simulink model "F16Block"  (R2017a)
settings: Solver=VariableStepAuto  StartTime=0.0  StopTime=400  FixedStep=delta_T  RelTol=1e-3  EnableMultiTasking=on
values from neighbouring files (symbols this model uses):
  trim_control = [xu(2);xu(4);xu(5)]    [trim_F16.m]
  trim_state = xu(1:12)    [trim_F16.m]
  trim_thrust = xu(13)    [trim_F16.m]
undefined symbols (not defined in the file or in its folder): DisAil_1, DisAil_2, DisAil_3, DisEle_1, DisEle_2, DisEle_3, DisRud_1, DisRud_2, DisRud_3, fi_flag_Simulink
libraries: F16_Actuator_Library x9
settings Model: ExtModeAutoUpdateStatusClock=off  Creator=keviczky  LastModifiedBy=wagneda1
settings DataIOCC: Decimation=50  SaveFormat=Array  SignalLoggingName=sigsOut
settings OptimizationCC: BooleanDataType=off
settings DebuggingCC: SaveWithParameterizedLinksMsg=none  UnderspecifiedInitializationDetection=Classic  MergeDetectMultiDrivingBlocksExec=none  SignalResolutionControl=TryResolveAllWithWarning  MultiTaskDSMMsg=warning  MultiTaskCondExecSysMsg=none
settings HardwareCC: ProdBitPerPointer=32  ProdBitPerSizeT=32  ProdBitPerPtrDiffT=32  ProdLargestAtomicFloat=None  ProdIntDivRoundTo=Undefined  ProdEndianess=Unspecified  ProdWordSize=32  ProdHWDeviceType=32-bit Generic  TargetUnknown=on
settings ModelReferenceCC: PropagateSignalLabelsOutOfModel=off
settings GRTTargetCC: TargetLangStandard=C89/C90 (ANSI)  CombineOutputUpdateFcns=off  GRTInterface=on
settings ConfigComp: CovMetricSettings=dw  CovHtmlReporting=on  CovSaveCumulativeToWorkspaceVar=on  CovSaveSingleToWorkspaceVar=on  CovExternalEMLEnable=off

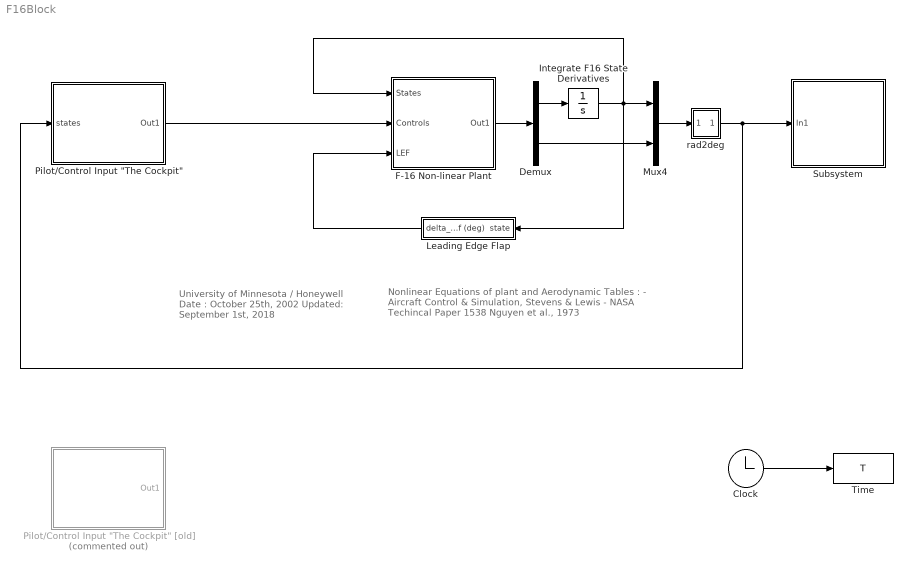
== system F16Block ==
  note: University of Minnesota / Honeywell
      | Date : October 25th, 2002
      | Updated: September 1st, 2018
  note: Nonlinear Equations of plant and Aerodynamic Tables :
      | - Aircraft Control & Simulation, Stevens & Lewis
      | - NASA Techincal Paper 1538 Nguyen et al., 1973
  Clock : Clock
      settings: Decimation=50
  Demux : Demux  Outputs=[12 6]
  F-16 Non-linear Plant : Subsystem
      mask Display: image('f16thumb.jpg')
  Integrate F16 State Derivatives : Integrator  InitialCondition=trim_state
  Leading Edge Flap : Subsystem
  Mux4 : Mux  Inputs=2
  "Pilot/Control Input \"The Cockpit\"" : Subsystem
      mask Display: image('f16cockpit.jpg')
  "Pilot/Control Input \"The Cockpit\" [old]" : Subsystem  Commented=on
      mask Display: image(imread('f16cockpit.jpg'))
  Subsystem : Subsystem
      mask Display: image('f16output.jpg')
  Time : ToWorkspace  VariableName=T  SampleTime=-1
      settings: Decimation=100
  rad2deg : Subsystem
  wires:
  Mux4/1 -> rad2deg/1(In1)
  Demux/1 -> Integrate F16 State Derivatives/1
  Demux/2 -> Mux4/2
  "Pilot/Control Input \"The Cockpit\""/1(Out1) -> F-16 Non-linear Plant/2(Controls)
  Leading Edge Flap/1(delta_lef (deg)) -> F-16 Non-linear Plant/3(LEF)
  F-16 Non-linear Plant/1(Out1) -> Demux/1
  Integrate F16 State Derivatives/1 -> Mux4/1, Leading Edge Flap/1(state), F-16 Non-linear Plant/1(States)
  Clock/1 -> Time/1
  rad2deg/1(Out1) -> "Pilot/Control Input \"The Cockpit\""/1(states), Subsystem/1(In1)

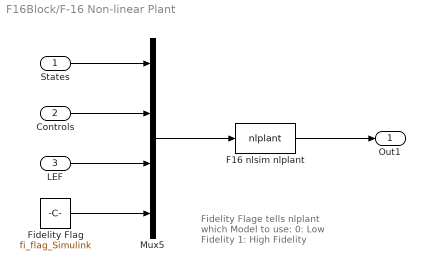
== system F16Block/F-16 Non-linear Plant ==
  note: Fidelity Flage tells nlplant
      | which Model to use:
      | 0: Low Fidelity
      | 1: High Fidelity
  States : Inport
  Controls : Inport  Port=2
  LEF : Inport  Port=3
  F16 nlsim nlplant : MATLABFcn  MATLABFcn=nlplant  OutputDimensions=18  OutputSignalType=real
  Fidelity Flag : Constant  Value=fi_flag_Simulink
  Mux5 : Mux  Inputs=[12 4 1 1]
  Out1 : Outport
  wires:
  Mux5/1 -> F16 nlsim nlplant/1
  F16 nlsim nlplant/1 -> Out1/1
  Fidelity Flag/1 -> Mux5/4
  LEF/1 -> Mux5/3
  Controls/1 -> Mux5/2
  States/1 -> Mux5/1

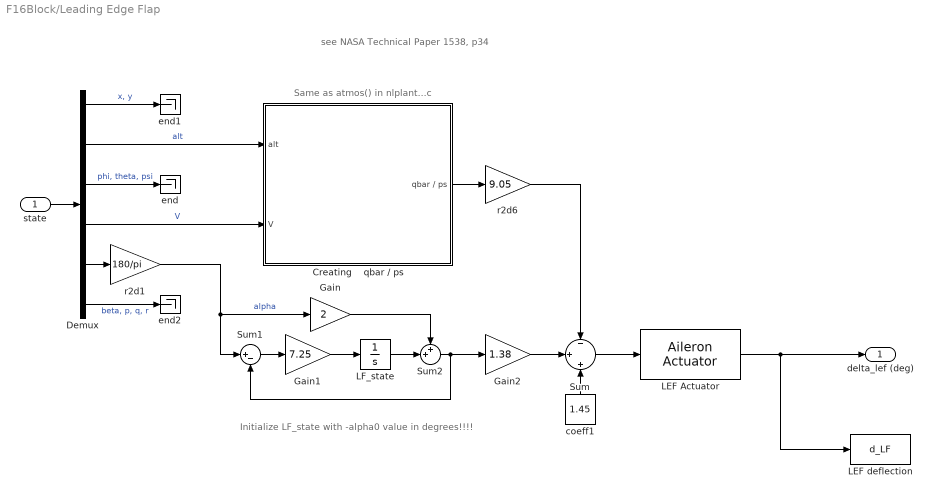
== system F16Block/Leading Edge Flap ==
  note: see NASA Technical Paper 1538, p34
  note: Same as atmos() in nlplant...c
  note: Initialize LF_state with -alpha0 value in degrees!!!!
  state : Inport
  Creating    qbar / ps : Subsystem
  Demux : Demux  Outputs=[2,1,3,1,1,4]
  Gain : Gain  Gain=2  SaturateOnIntegerOverflow=on  OutDataTypeStr=Inherit: Same as input  ParamDataTypeStr=Inherit: Same as input
  Gain1 : Gain  Gain=7.25  SaturateOnIntegerOverflow=on  OutDataTypeStr=Inherit: Same as input  ParamDataTypeStr=Inherit: Same as input
  Gain2 : Gain  Gain=1.38  SaturateOnIntegerOverflow=on  OutDataTypeStr=Inherit: Same as input  ParamDataTypeStr=Inherit: Same as input
  LEF Actuator : F16_Actuator_Library/Aileron Actuator
      link override Command Saturation: UpperLimit=25  LowerLimit=0
      link override Gain: Gain=1/0.136
      link override "Integrator ": InitialCondition=dLEF
      link override Rate Saturation: UpperLimit=25  LowerLimit=-25
  LEF deflection : ToWorkspace  VariableName=d_LF  SampleTime=-1
      settings: Decimation=100
  LF_state : Integrator  InitialCondition=-trim_state(8)*180/pi
  Sum : Sum  Inputs=-|+|+  SaturateOnIntegerOverflow=on  InputSameDT=on  OutDataTypeStr=Inherit: Same as first input
  Sum1 : Sum  Inputs=|+-  SaturateOnIntegerOverflow=on  InputSameDT=on  OutDataTypeStr=Inherit: Same as first input
  Sum2 : Sum  Inputs=++|  SaturateOnIntegerOverflow=on  InputSameDT=on  OutDataTypeStr=Inherit: Same as first input
  coeff1 : Constant  Value=1.45
  end : Terminator
  end1 : Terminator
  end2 : Terminator
  r2d1 : Gain  Gain=180/pi  SaturateOnIntegerOverflow=on  OutDataTypeStr=Inherit: Same as input  ParamDataTypeStr=Inherit: Same as input
  r2d6 : Gain  Gain=9.05  SaturateOnIntegerOverflow=on  OutDataTypeStr=Inherit: Same as input  ParamDataTypeStr=Inherit: Same as input
  delta_lef (deg) : Outport
  wires:
  LEF Actuator/1 -> LEF deflection/1, delta_lef (deg)/1
  Sum/1 -> LEF Actuator/1
  Demux/3 -> end/1  "phi, theta, psi"
  state/1 -> Demux/1
  Sum1/1 -> Gain1/1
  Gain1/1 -> LF_state/1
  Gain/1 -> Sum2/1
  Gain2/1 -> Sum/2
  Demux/1 -> end1/1  "x, y"
  Demux/5 -> r2d1/1
  Demux/6 -> end2/1  "beta, p, q, r"
  coeff1/1 -> Sum/3
  Sum2/1 -> Sum1/2, Gain2/1
  LF_state/1 -> Sum2/2
  r2d1/1 -> Sum1/1, Gain/1  "alpha"
  Demux/4 -> Creating    qbar / ps/2(V)  "V"
  Creating    qbar / ps/1(qbar / ps) -> r2d6/1
  r2d6/1 -> Sum/1
  Demux/2 -> Creating    qbar / ps/1(alt)  "alt"

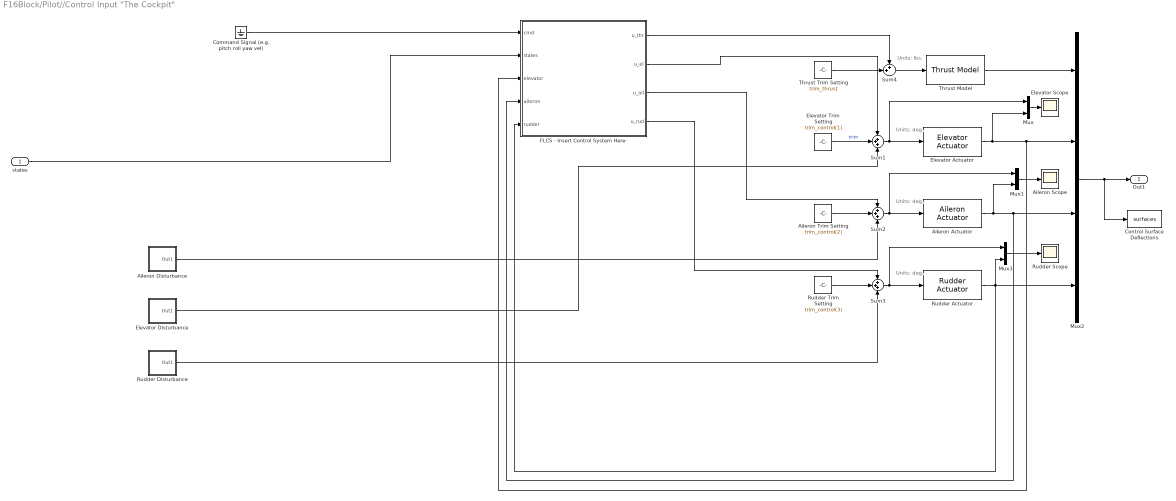
== system F16Block/Pilot//Control Input "The Cockpit" ==
  note: Units: lbs.
  note: Units: deg.
  note: Units: deg.
  note: Units: deg.
  states : Inport
  Aileron Actuator : F16_Actuator_Library/Aileron Actuator
  Aileron Scope : Scope
  Aileron Disturbance : Subsystem
  Aileron Trim Setting : Constant  Value=trim_control(2)
  Command Signal (e.g. pitch roll yaw vel) : Ground
  Control Surface Deflections : ToWorkspace  VariableName=surfaces  SampleTime=-1
      settings: Decimation=100
  Elevator Actuator : F16_Actuator_Library/Elevator Actuator
  Elevator Scope : Scope
  Elevator Disturbance : Subsystem
  Elevator Trim Setting : Constant  Value=trim_control(1)  VectorParams1D=off
  FLCS - Insert Control System Here- : Subsystem
  Mux : Mux  Inputs=2
  Mux1 : Mux  Inputs=2
  Mux2 : Mux
  Mux3 : Mux  Inputs=2
  Rudder Actuator : F16_Actuator_Library/Rudder Actuator
  Rudder Scope : Scope
  Rudder Disturbance : Subsystem
  Rudder Trim Setting : Constant  Value=trim_control(3)
  Sum1 : Sum  Inputs=+++  SaturateOnIntegerOverflow=on  InputSameDT=on  OutDataTypeStr=Inherit: Same as first input
  Sum2 : Sum  Inputs=+++  SaturateOnIntegerOverflow=on  InputSameDT=on  OutDataTypeStr=Inherit: Same as first input
  Sum3 : Sum  Inputs=+++  SaturateOnIntegerOverflow=on  InputSameDT=on  OutDataTypeStr=Inherit: Same as first input
  Sum4 : Sum  Inputs=++|  SaturateOnIntegerOverflow=on  InputSameDT=on  OutDataTypeStr=Inherit: Same as first input
  Thrust Model : F16_Actuator_Library/Thrust Model
  Thrust Trim Setting : Constant  Value=trim_thrust
  Out1 : Outport
  wires:
  Thrust Model/1 -> Mux2/1
  Sum1/1 -> Mux/1, Elevator Actuator/1
  Elevator Trim Setting/1 -> Sum1/2  "trim"
  Sum2/1 -> Mux1/1, Aileron Actuator/1
  Aileron Trim Setting/1 -> Sum2/2
  Sum3/1 -> Mux3/1, Rudder Actuator/1
  Rudder Trim Setting/1 -> Sum3/2
  Mux2/1 -> Out1/1, Control Surface Deflections/1
  Elevator Actuator/1 -> FLCS - Insert Control System Here-/3(elevator), Mux2/2, Mux/2
  Aileron Actuator/1 -> FLCS - Insert Control System Here-/4(aileron), Mux2/3, Mux1/2
  Rudder Actuator/1 -> Mux2/4, Mux3/2, FLCS - Insert Control System Here-/5(rudder)
  Mux/1 -> Elevator Scope/1
  Mux1/1 -> Aileron Scope/1
  Mux3/1 -> Rudder Scope/1
  Sum4/1 -> Thrust Model/1
  Thrust Trim Setting/1 -> Sum4/2
  Elevator Disturbance/1(Out1) -> Sum1/3
  Aileron Disturbance/1(Out1) -> Sum2/3
  Rudder Disturbance/1(Out1) -> Sum3/3
  states/1 -> FLCS - Insert Control System Here-/2(states)
  Command Signal (e.g. pitch roll yaw vel)/1 -> FLCS - Insert Control System Here-/1(cmd)
  FLCS - Insert Control System Here-/1(u_thr) -> Sum4/1
  FLCS - Insert Control System Here-/2(u_el) -> Sum1/1
  FLCS - Insert Control System Here-/3(u_ail) -> Sum2/1
  FLCS - Insert Control System Here-/4(u_rud) -> Sum3/1

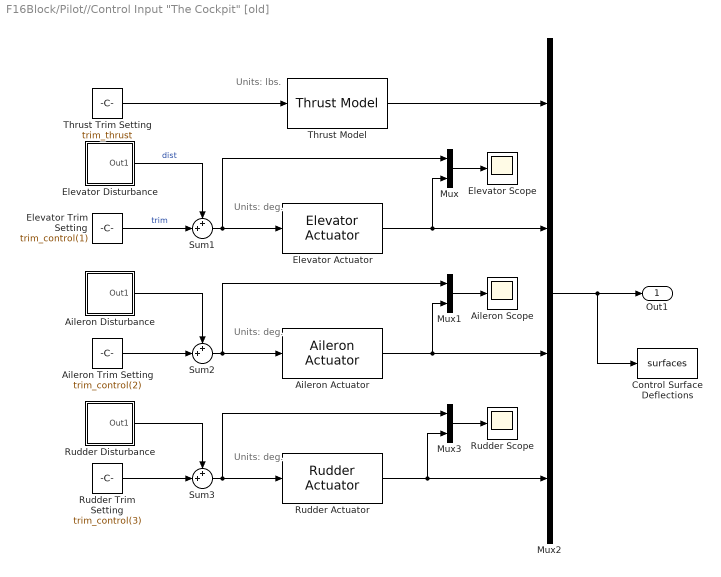
== system F16Block/Pilot//Control Input "The Cockpit" [old] ==
  note: Units: lbs.
  note: Units: deg.
  note: Units: deg.
  note: Units: deg.
  Aileron Actuator : F16_Actuator_Library/Aileron Actuator
  Aileron Scope : Scope
  Aileron Disturbance : Subsystem
  Aileron Trim Setting : Constant  Value=trim_control(2)
  Control Surface Deflections : ToWorkspace  VariableName=surfaces  SampleTime=-1
      settings: Decimation=100
  Elevator Actuator : F16_Actuator_Library/Elevator Actuator
  Elevator Scope : Scope
  Elevator Disturbance : Subsystem
  Elevator Trim Setting : Constant  Value=trim_control(1)  VectorParams1D=off
  Mux : Mux  Inputs=2
  Mux1 : Mux  Inputs=2
  Mux2 : Mux
  Mux3 : Mux  Inputs=2
  Rudder Actuator : F16_Actuator_Library/Rudder Actuator
  Rudder Scope : Scope
  Rudder Disturbance : Subsystem
  Rudder Trim Setting : Constant  Value=trim_control(3)
  Sum1 : Sum  Inputs=++|  SaturateOnIntegerOverflow=on  InputSameDT=on  OutDataTypeStr=Inherit: Same as first input
  Sum2 : Sum  Inputs=++|  SaturateOnIntegerOverflow=on  InputSameDT=on  OutDataTypeStr=Inherit: Same as first input
  Sum3 : Sum  Inputs=++|  SaturateOnIntegerOverflow=on  InputSameDT=on  OutDataTypeStr=Inherit: Same as first input
  Thrust Model : F16_Actuator_Library/Thrust Model
  Thrust Trim Setting : Constant  Value=trim_thrust
  Out1 : Outport
  wires:
  Thrust Model/1 -> Mux2/1
  Sum1/1 -> Mux/1, Elevator Actuator/1
  Elevator Trim Setting/1 -> Sum1/2  "trim"
  Sum2/1 -> Mux1/1, Aileron Actuator/1
  Aileron Trim Setting/1 -> Sum2/2
  Aileron Disturbance/1(Out1) -> Sum2/1
  Elevator Disturbance/1(Out1) -> Sum1/1  "dist"
  Sum3/1 -> Mux3/1, Rudder Actuator/1
  Rudder Disturbance/1(Out1) -> Sum3/1
  Rudder Trim Setting/1 -> Sum3/2
  Mux2/1 -> Out1/1, Control Surface Deflections/1
  Elevator Actuator/1 -> Mux2/2, Mux/2
  Aileron Actuator/1 -> Mux2/3, Mux1/2
  Rudder Actuator/1 -> Mux2/4, Mux3/2
  Mux/1 -> Elevator Scope/1
  Mux1/1 -> Aileron Scope/1
  Mux3/1 -> Rudder Scope/1
  Thrust Trim Setting/1 -> Thrust Model/1

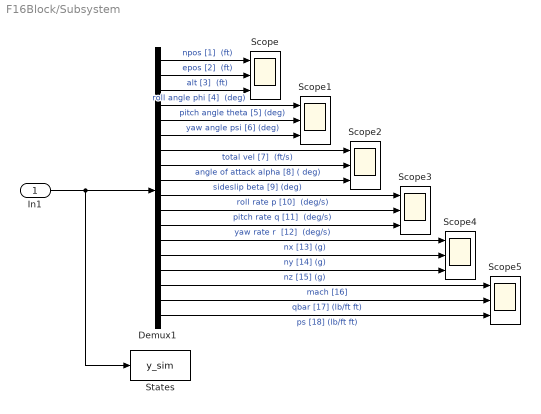
== system F16Block/Subsystem ==
  In1 : Inport
  Demux1 : Demux  Outputs=18
  Scope{,1..5} (6 alike) : Scope  NumInputPorts=3
  States : ToWorkspace  VariableName=y_sim  SampleTime=-1
      settings: Decimation=100
  wires:
  Demux1/1 -> Scope/1  "npos [1]  (ft)"
  Demux1/2 -> Scope/2  "epos [2]  (ft)"
  Demux1/3 -> Scope/3  "alt [3]  (ft)"
  Demux1/5 -> Scope1/2  "pitch angle theta [5] (deg)"
  Demux1/6 -> Scope1/3  "yaw angle psi [6] (deg)"
  Demux1/7 -> Scope2/1  "total vel [7]  (ft/s)"
  Demux1/8 -> Scope2/2  "angle of attack alpha [8] ( deg)"
  Demux1/9 -> Scope2/3  "sideslip beta [9] (deg)"
  Demux1/10 -> Scope3/1  "roll rate p [10]  (deg/s)"
  Demux1/11 -> Scope3/2  "pitch rate q [11]  (deg/s)"
  Demux1/12 -> Scope3/3  "yaw rate r  [12]  (deg/s)"
  Demux1/13 -> Scope4/1  "nx [13] (g)"
  Demux1/14 -> Scope4/2  "ny [14] (g)"
  Demux1/15 -> Scope4/3  "nz [15] (g)"
  Demux1/4 -> Scope1/1  "roll angle phi [4]  (deg)"
  Demux1/16 -> Scope5/1  "mach [16]"
  Demux1/17 -> Scope5/2  "qbar [17] (lb/ft ft)"
  Demux1/18 -> Scope5/3  "ps [18] (lb/ft ft)"
  In1/1 -> Demux1/1, States/1

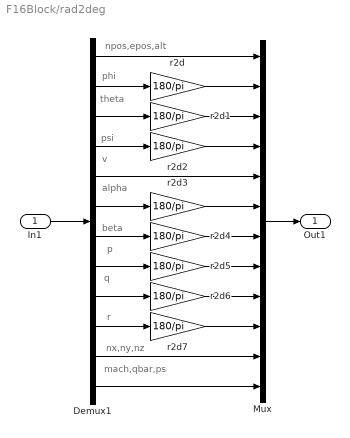
== system F16Block/rad2deg ==
  note: npos,epos,alt
  note: phi
  note: theta
  note: psi
  note: v
  note: alpha
  note: beta
  note: p
  note: q
  note: r
  note: nx,ny,nz
  note: mach,qbar,ps
  In1 : Inport
  Demux1 : Demux  Outputs=[3 1 1 1 1 1 1 1 1 1 3 3]
  Mux : Mux  Inputs=[3 1 1 1 1 1 1 1 1 1 3 3]
  r2d{,1..7} (8 alike) : Gain  Gain=180/pi  SaturateOnIntegerOverflow=on  OutDataTypeStr=Inherit: Same as input  ParamDataTypeStr=Inherit: Same as input
  Out1 : Outport
  wires:
  In1/1 -> Demux1/1
  Demux1/2 -> r2d/1
  Demux1/3 -> r2d1/1
  Demux1/4 -> r2d2/1
  Demux1/1 -> Mux/1
  Demux1/5 -> Mux/5
  r2d2/1 -> Mux/4
  r2d1/1 -> Mux/3
  r2d/1 -> Mux/2
  Demux1/6 -> r2d3/1
  Demux1/7 -> r2d4/1
  Demux1/8 -> r2d5/1
  Demux1/9 -> r2d6/1
  Demux1/10 -> r2d7/1
  r2d4/1 -> Mux/7
  r2d5/1 -> Mux/8
  r2d6/1 -> Mux/9
  r2d7/1 -> Mux/10
  Mux/1 -> Out1/1
  Demux1/11 -> Mux/11
  Demux1/12 -> Mux/12
  r2d3/1 -> Mux/6

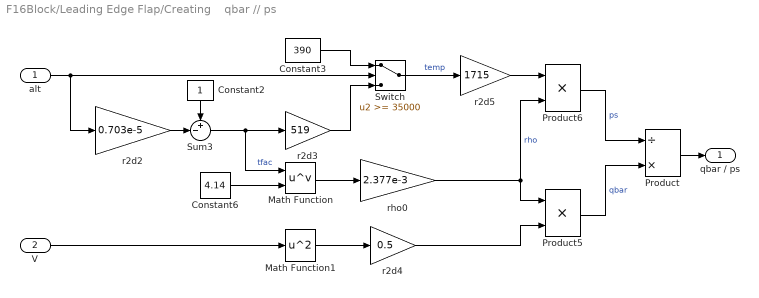
== system F16Block/Leading Edge Flap/Creating    qbar // ps ==
  alt : Inport
  V : Inport  Port=2
  Constant2 : Constant
  Constant3 : Constant  Value=390
  Constant6 : Constant  Value=4.14
  Math Function : Math  Operator=pow  SaturateOnIntegerOverflow=on
  Math Function1 : Math  Operator=square  SaturateOnIntegerOverflow=on
  Product : Product  Inputs=/*  SaturateOnIntegerOverflow=on  InputSameDT=on  OutDataTypeStr=Inherit: Same as first input
  Product5 : Product  Inputs=**  SaturateOnIntegerOverflow=on  InputSameDT=on  OutDataTypeStr=Inherit: Same as first input
  Product6 : Product  Inputs=**  SaturateOnIntegerOverflow=on  InputSameDT=on  OutDataTypeStr=Inherit: Same as first input
  Sum3 : Sum  Inputs=+-|  SaturateOnIntegerOverflow=on  InputSameDT=on  OutDataTypeStr=Inherit: Same as first input
  Switch : Switch  Threshold=35000  SaturateOnIntegerOverflow=on  InputSameDT=on
  r2d2 : Gain  Gain=0.703e-5  SaturateOnIntegerOverflow=on  OutDataTypeStr=Inherit: Same as input  ParamDataTypeStr=Inherit: Same as input
  r2d3 : Gain  Gain=519  SaturateOnIntegerOverflow=on  OutDataTypeStr=Inherit: Same as input  ParamDataTypeStr=Inherit: Same as input
  r2d4 : Gain  Gain=0.5  SaturateOnIntegerOverflow=on  OutDataTypeStr=Inherit: Same as input  ParamDataTypeStr=Inherit: Same as input
  r2d5 : Gain  Gain=1715  SaturateOnIntegerOverflow=on  OutDataTypeStr=Inherit: Same as input  ParamDataTypeStr=Inherit: Same as input
  rho0 : Gain  Gain=2.377e-3  SaturateOnIntegerOverflow=on  OutDataTypeStr=Inherit: Same as input  ParamDataTypeStr=Inherit: Same as input
  qbar / ps : Outport
  wires:
  alt/1 -> r2d2/1, Switch/2
  Sum3/1 -> Math Function/1, r2d3/1  "tfac"
  Constant3/1 -> Switch/1
  r2d3/1 -> Switch/3
  Constant6/1 -> Math Function/2
  rho0/1 -> Product5/1, Product6/2  "rho"
  Math Function1/1 -> r2d4/1
  r2d2/1 -> Sum3/2
  Constant2/1 -> Sum3/1
  Math Function/1 -> rho0/1
  r2d4/1 -> Product5/2
  Switch/1 -> r2d5/1  "temp"
  r2d5/1 -> Product6/1
  Product6/1 -> Product/1  "ps"
  Product5/1 -> Product/2  "qbar"
  Product/1 -> qbar / ps/1
  V/1 -> Math Function1/1

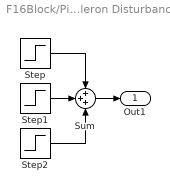
== system F16Block/Pilot//Control Input "The Cockpit"/Aileron Disturbance ==
  Step : Step  After=DisAil_1  SampleTime=0
  Step1 : Step  Time=3  After=DisAil_2  SampleTime=0
  Step2 : Step  Time=5  After=DisAil_3  SampleTime=0
  Sum : Sum  Inputs=+++  SaturateOnIntegerOverflow=on  InputSameDT=on  OutDataTypeStr=Inherit: Same as first input
  Out1 : Outport
  wires:
  Step1/1 -> Sum/2
  Step/1 -> Sum/1
  Step2/1 -> Sum/3
  Sum/1 -> Out1/1

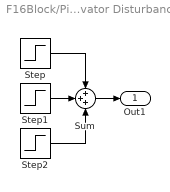
== system F16Block/Pilot//Control Input "The Cockpit"/Elevator Disturbance ==
  Step : Step  After=DisEle_1  SampleTime=0
  Step1 : Step  Time=3  After=DisEle_2  SampleTime=0
  Step2 : Step  Time=5  After=DisEle_3  SampleTime=0
  Sum : Sum  Inputs=+++  SaturateOnIntegerOverflow=on  InputSameDT=on  OutDataTypeStr=Inherit: Same as first input
  Out1 : Outport
  wires:
  Step1/1 -> Sum/2
  Step/1 -> Sum/1
  Step2/1 -> Sum/3
  Sum/1 -> Out1/1

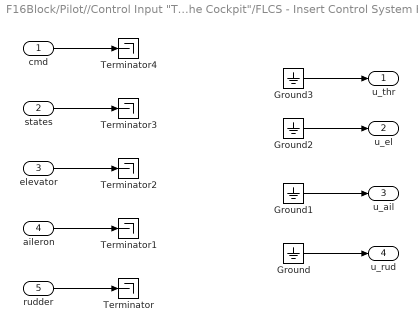
== system F16Block/Pilot//Control Input "The Cockpit"/FLCS - Insert Control System Here- ==
  cmd : Inport
  states : Inport  Port=2
  elevator : Inport  Port=3
  aileron : Inport  Port=4
  rudder : Inport  Port=5
  Ground{,1..3} (4 alike) : Ground
  Terminator{,1..4} (5 alike) : Terminator
  u_thr : Outport
  u_el : Outport  Port=2
  u_ail : Outport  Port=3
  u_rud : Outport  Port=4
  wires:
  Ground/1 -> u_rud/1
  Ground1/1 -> u_ail/1
  Ground2/1 -> u_el/1
  Ground3/1 -> u_thr/1
  rudder/1 -> Terminator/1
  aileron/1 -> Terminator1/1
  elevator/1 -> Terminator2/1
  states/1 -> Terminator3/1
  cmd/1 -> Terminator4/1

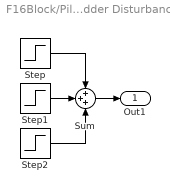
== system F16Block/Pilot//Control Input "The Cockpit"/Rudder Disturbance ==
  Step : Step  After=DisRud_1  SampleTime=0
  Step1 : Step  Time=3  After=DisRud_2  SampleTime=0
  Step2 : Step  Time=5  After=DisRud_3  SampleTime=0
  Sum : Sum  Inputs=+++  SaturateOnIntegerOverflow=on  InputSameDT=on  OutDataTypeStr=Inherit: Same as first input
  Out1 : Outport
  wires:
  Step1/1 -> Sum/2
  Step/1 -> Sum/1
  Step2/1 -> Sum/3
  Sum/1 -> Out1/1

== system F16Block/Pilot//Control Input "The Cockpit" [old]/Aileron Disturbance ==
  Step : Step  After=DisAil_1  SampleTime=0
  Step1 : Step  Time=3  After=DisAil_2  SampleTime=0
  Step2 : Step  Time=5  After=DisAil_3  SampleTime=0
  Sum : Sum  Inputs=+++  SaturateOnIntegerOverflow=on  InputSameDT=on  OutDataTypeStr=Inherit: Same as first input
  Out1 : Outport
  wires:
  Step1/1 -> Sum/2
  Step/1 -> Sum/1
  Step2/1 -> Sum/3
  Sum/1 -> Out1/1

== system F16Block/Pilot//Control Input "The Cockpit" [old]/Elevator Disturbance ==
  Step : Step  After=DisEle_1  SampleTime=0
  Step1 : Step  Time=3  After=DisEle_2  SampleTime=0
  Step2 : Step  Time=5  After=DisEle_3  SampleTime=0
  Sum : Sum  Inputs=+++  SaturateOnIntegerOverflow=on  InputSameDT=on  OutDataTypeStr=Inherit: Same as first input
  Out1 : Outport
  wires:
  Step1/1 -> Sum/2
  Step/1 -> Sum/1
  Step2/1 -> Sum/3
  Sum/1 -> Out1/1

== system F16Block/Pilot//Control Input "The Cockpit" [old]/Rudder Disturbance ==
  Step : Step  After=DisRud_1  SampleTime=0
  Step1 : Step  Time=3  After=DisRud_2  SampleTime=0
  Step2 : Step  Time=5  After=DisRud_3  SampleTime=0
  Sum : Sum  Inputs=+++  SaturateOnIntegerOverflow=on  InputSameDT=on  OutDataTypeStr=Inherit: Same as first input
  Out1 : Outport
  wires:
  Step1/1 -> Sum/2
  Step/1 -> Sum/1
  Step2/1 -> Sum/3
  Sum/1 -> Out1/1
